simulink model "Reactor"  (R2023a)
settings: Solver=VariableStepAuto  StartTime=0.0  StopTime=20  RelTol=1e-3
values from neighbouring files (symbols this model uses):
  k = 50    [constants.m]
  q = 0.25    [constants.m]
  V = 10    [constants.m]
settings Model: Creator=Researcher  LastModifiedBy=Researcher

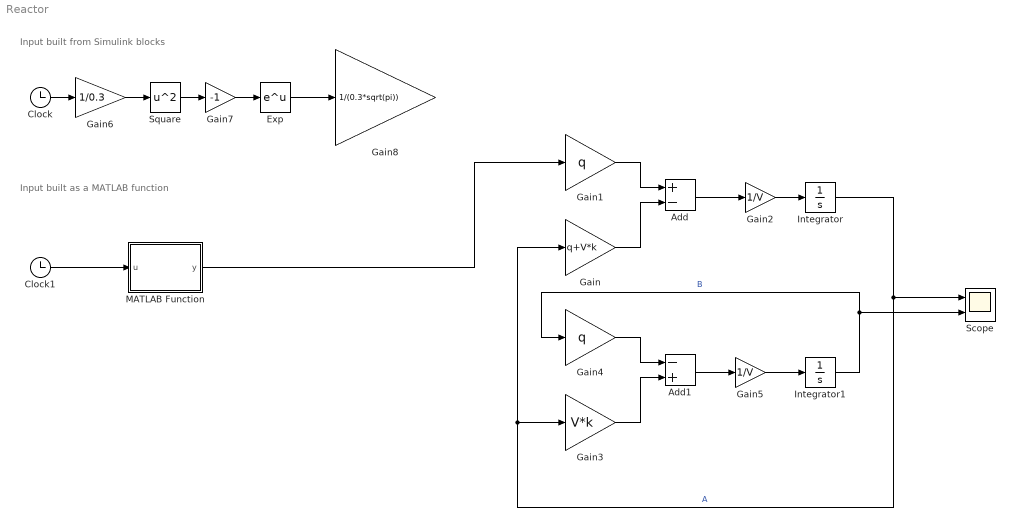
== system Reactor ==
  note: Input built as a MATLAB function
  note: Input built from Simulink blocks
  Add : Sum  Inputs=+-
  Add1 : Sum  Inputs=-+
  Clock : Clock
  Clock1 : Clock
  Exp : Math
  Gain : Gain  Gain=q+V*k
  Gain1 : Gain  Gain=q
  Gain2 : Gain  Gain=1/V
  Gain3 : Gain  Gain=V*k
  Gain4 : Gain  Gain=q
  Gain5 : Gain  Gain=1/V
  Gain6 : Gain  Gain=1/0.3
  Gain7 : Gain  Gain=-1
  Gain8 : Gain  Gain=1/(0.3*sqrt(pi))
  Integrator : Integrator
  Integrator1 : Integrator
  MATLAB Function : MATLAB Function  TreatAsAtomicUnit=on
  Scope : Scope  NumInputPorts=2
  Square : Math  Operator=square
  wires:
  Integrator/1 -> Scope/1, Gain/1, Gain3/1  "A"
  Gain1/1 -> Add/1
  Gain/1 -> Add/2
  Add/1 -> Gain2/1
  Gain2/1 -> Integrator/1
  Gain5/1 -> Integrator1/1
  Gain3/1 -> Add1/2
  Gain4/1 -> Add1/1
  Add1/1 -> Gain5/1
  Integrator1/1 -> Scope/2, Gain4/1  "B"
  Clock/1 -> Gain6/1
  Gain6/1 -> Square/1
  Square/1 -> Gain7/1
  Gain7/1 -> Exp/1
  Exp/1 -> Gain8/1
  Clock1/1 -> MATLAB Function/1(u)
  MATLAB Function/1(y) -> Gain1/1

== matlab function Reactor/MATLAB Function ==
  data: u input; y output
function y = fcn(u)

y = (1/(0.3*sqrt(pi)))*exp(-((u/0.3)^2));
% y = u;
